simulink model "sinkTCP"  (R2021b)
settings: Solver=FixedStepAuto  StartTime=0.0  StopTime=10.0  RelTol=1e-3
undefined symbols (not defined in the file or in its folder): SampleTime
libraries: instrumentlib x1
settings Model: DataDictionary=theSystem.sldd  Creator=samwarner  LastModifiedBy=samwarner

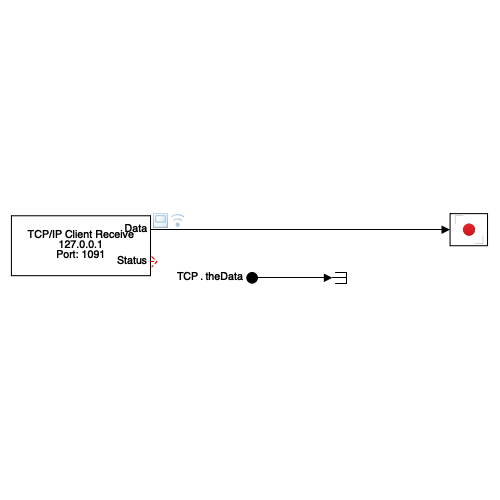
[thumbnail: Simulink's stored preview of the top-level diagram]
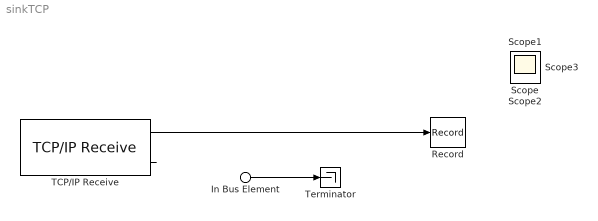
== system sinkTCP ==
  In Bus Element : Inport  PortName=TCP  Element=theData
  Record : Record  RecordToFile=on  FileSettingsInternal="{\"entries\":[{\"content\":{\"excelSettings\":{\"content\":{},\"type\":\"Streamout.ExcelSettings\"}},\"type\":\"Streamout.FileSettingStorage\",\"uuid\":\"3b51fcac-aedc-48a9-bcd0-f1828d056c64\"}],\"packageUris\":[\"http://schema.mathworks.com/mf0/streamout_blocks/R2020a\"],\"version\":\"1.0\"}"  SignalsInternal="{\"entries\":[{\"content\":{\"signals\":[{\"content\":{\"blockPath\":[\"sinkTCP/Record\"],\"channel\":[],\"dimensions\":[1],\"domain\":\"sinkTCP/Record\",\"lineColor\":\"#edb120\",\"plots\":[1],\"port\":1,\"sid\":[],\"signalID\":9,\"signalName\":\"<theDaata>\"},\"type\":\"RecordBlkView.Signal\",\"uuid\":\"9c0d2a86-bc90-4d2e-8cdd-f0a603cc96a9\"}]},\"type\":\"RecordBlkView.InputSignals\",\"uuid\":\"e6f81dbd-277e-4fcd-ba59-1d3f58789b7c\"},{\"content\":{\"signals\":[{\"content\":{\"blockPath\":[\"sinkTCP/Record\"],\"channel\":[],\"dimensions\":[1],\"domain\":\"sinkTCP/Record\",\"lineColor\":\"#edb120\",\"plots\":[],\"port\":1,\"sid\":[],\"signalID\":9,\"signalName\":\"<theDaata>\"},\"type\":\"RecordBlkView.Signal\",\"uuid\":\"41a97796-8587-4255-bc15-999938db6bb8\"}]},\"type\":\"RecordBlkView.InputSignals\",\"uuid\":\"34b84d9d-0be9-4186-acc1-1427aacb70e6\"}],\"packageUris\":[\"http://schema.mathworks.com/mf0/streamout_blocks/R2020a\"],\"version\":\"1.0\"}"  VisualizationBindings="{\"sparklinesplugin\":{\"info\":[{\"bindingParametersList\":[],\"subplotID\":1}]}}"
  TCP/IP Receive : instrumentlib/TCP//IP Receive  Host=127.0.0.1  Port=1091  DataSize=1  DataType=uint8  ASCIIFormatting=%f  Terminator=LF  CustomTerminator=10  ByteOrder=big-endian  EnableBlockingMode=off  Timeout=10  SampleTime=SampleTime  SimulateUsing=Interpreted execution
  Terminator : Terminator
  Scope{,1..3} (4 alike) : Scope
  wires:
  TCP/IP Receive/1 -> Record/1
  In Bus Element/1 -> Terminator/1
  TCP/IP Receive/2 -> ?
